simulink model "ES106A_StHlthSigStc"  (R2013b)
settings: Solver=FixedStepDiscrete  SolverMode=SingleTasking  StartTime=0.0  StopTime=1  FixedStep=0.002  RelTol=1e-3
values from neighbouring files (symbols this model uses):
  APPL10_CNT_U08 = DataDict.Constant    [ES106A_StHlthSigStc_DataDict.m]
  BITSPERBYTE_CNT_U08 = DataDict.Constant    [ES106A_StHlthSigStc_DataDict.m]
  ENOTOK_CNT_U08 = DataDict.Constant    [ES106A_StHlthSigStc_DataDict.m]
  EOK_CNT_U08 = DataDict.Constant    [ES106A_StHlthSigStc_DataDict.m]
  LOWRMASKVAL_CNT_U32 = DataDict.Constant    [ES106A_StHlthSigStc_DataDict.m]
  NROFCRCAREA_CNT_U08 = DataDict.ConfigParam    [ES106A_StHlthSigStc_DataDict.m]
  NVMAVRGPOSN_CNT_U08 = DataDict.Constant    [ES106A_StHlthSigStc_DataDict.m]
  NVMMAXPOSN_CNT_U08 = DataDict.Constant    [ES106A_StHlthSigStc_DataDict.m]
  NVMMINPOSN_CNT_U08 = DataDict.Constant    [ES106A_StHlthSigStc_DataDict.m]
  NVMSAMPLECNTRPOSN_CNT_U08 = DataDict.Constant    [ES106A_StHlthSigStc_DataDict.m]
  RAMAVRGPOSN_CNT_U08 = DataDict.Constant    [ES106A_StHlthSigStc_DataDict.m]
  RAMMAXPOSN_CNT_U08 = DataDict.Constant    [ES106A_StHlthSigStc_DataDict.m]
  RAMMINPOSN_CNT_U08 = DataDict.Constant    [ES106A_StHlthSigStc_DataDict.m]
  RAMRAWPOSN_CNT_U08 = DataDict.Constant    [ES106A_StHlthSigStc_DataDict.m]
  SIGCNT_ULS_U08 = DataDict.ConfigParam    [ES106A_StHlthSigStc_DataDict.m]
  SigStcPrmInst = DataDict.PIM    [ES106A_StHlthSigStc_DataDict.m]
  STHLTHMAXVAL_CNT_U08 = DataDict.Constant    [ES106A_StHlthSigStc_DataDict.m]
  WORDSIZE_CNT_U08 = DataDict.Constant    [ES106A_StHlthSigStc_DataDict.m]
undefined symbols (not defined in the file or in its folder): NvmGetErrSts1, StHlthTaskRef1
libraries: simulink x37, NxtrNvM x4, NxtrMax x4, NxtrMin x4
(part 5 of 5)

== system ES106A_StHlthSigStc/StHlthSigStc/StHlthStcPwrDwn/For Iterator Subsystem/If Action Subsystem/Statistical data computation for Controller Life Cycle/While Iterator Subsystem/Switch Case Action Subsystem ==
  In1 : Inport
  Action Port : ActionPort  ActionType=case
  CopyRight2 : Subsystem  Description=|  mask(Copyright Information){none=on}
      | Copyright info block.                                               
      |                                                                     
      | Place copyright information at the top of every subsystem in design.
      mask prompts: none "No parameters"
      mask help: Place copyright information at the top of every subsystem in design.
      mask Display:
      | NxtrConf = 'Nexteer Confidential';
      | 
      | sys = bdroot; %handle for the current model ("system")
      | first = get_param(sys,'Created');
      | if(isempty(first))
      |     first = datestr(now,'yyyy');
      | else
      |     first = first(end-3:end);  %year is last four digits
      | end
      | 
      | last = get_param(sys,'LastModifiedDate');
      | if isempty(last)
      |     last = datestr(now,'yyyy');
      | else
      |     last = last(end-3:end);
      | end
      | 
      | if strcmp(first,last)
      |     fprintf('%s -- Copyright %s Nexteer',NxtrConf,first)
      | else
      |     fprintf('%s -- %s%s- %s Nexteer',NxtrConf,char(169),first,last)
      | end
  Data Type Conversion : DataTypeConversion  OutDataTypeStr=uint32
  Shift Arithmetic3 : ArithShift  BitShiftNumber=SHIFTFAC24_ULS_U08  BitShiftDirection=Left
  Out1 : Outport
  wires:
  In1/1 -> Data Type Conversion/1
  Data Type Conversion/1 -> Shift Arithmetic3/1
  Shift Arithmetic3/1 -> Out1/1

== system ES106A_StHlthSigStc/StHlthSigStc/StHlthStcPwrDwn/For Iterator Subsystem/If Action Subsystem/Statistical data computation for Controller Life Cycle/While Iterator Subsystem/Switch Case Action Subsystem1 ==
  In1 : Inport
  Action Port : ActionPort  ActionType=case
  CopyRight2 : Subsystem  Description=|  mask(Copyright Information){none=on}
      | Copyright info block.                                               
      |                                                                     
      | Place copyright information at the top of every subsystem in design.
      mask prompts: none "No parameters"
      mask help: Place copyright information at the top of every subsystem in design.
      mask Display:
      | NxtrConf = 'Nexteer Confidential';
      | 
      | sys = bdroot; %handle for the current model ("system")
      | first = get_param(sys,'Created');
      | if(isempty(first))
      |     first = datestr(now,'yyyy');
      | else
      |     first = first(end-3:end);  %year is last four digits
      | end
      | 
      | last = get_param(sys,'LastModifiedDate');
      | if isempty(last)
      |     last = datestr(now,'yyyy');
      | else
      |     last = last(end-3:end);
      | end
      | 
      | if strcmp(first,last)
      |     fprintf('%s -- Copyright %s Nexteer',NxtrConf,first)
      | else
      |     fprintf('%s -- %s%s- %s Nexteer',NxtrConf,char(169),first,last)
      | end
  Data Type Conversion1 : DataTypeConversion  OutDataTypeStr=uint32
  Shift Arithmetic1 : ArithShift  BitShiftNumber=SHIFTFAC16_ULS_U08  BitShiftDirection=Left
  Out1 : Outport
  wires:
  In1/1 -> Data Type Conversion1/1
  Shift Arithmetic1/1 -> Out1/1
  Data Type Conversion1/1 -> Shift Arithmetic1/1

== system ES106A_StHlthSigStc/StHlthSigStc/StHlthStcPwrDwn/For Iterator Subsystem/If Action Subsystem/Statistical data computation for Controller Life Cycle/While Iterator Subsystem/Switch Case Action Subsystem2 ==
  In1 : Inport
  Action Port : ActionPort  ActionType=case
  CopyRight2 : Subsystem  Description=|  mask(Copyright Information){none=on}
      | Copyright info block.                                               
      |                                                                     
      | Place copyright information at the top of every subsystem in design.
      mask prompts: none "No parameters"
      mask help: Place copyright information at the top of every subsystem in design.
      mask Display:
      | NxtrConf = 'Nexteer Confidential';
      | 
      | sys = bdroot; %handle for the current model ("system")
      | first = get_param(sys,'Created');
      | if(isempty(first))
      |     first = datestr(now,'yyyy');
      | else
      |     first = first(end-3:end);  %year is last four digits
      | end
      | 
      | last = get_param(sys,'LastModifiedDate');
      | if isempty(last)
      |     last = datestr(now,'yyyy');
      | else
      |     last = last(end-3:end);
      | end
      | 
      | if strcmp(first,last)
      |     fprintf('%s -- Copyright %s Nexteer',NxtrConf,first)
      | else
      |     fprintf('%s -- %s%s- %s Nexteer',NxtrConf,char(169),first,last)
      | end
  Data Type Conversion1 : DataTypeConversion  OutDataTypeStr=uint32
  Shift Arithmetic2 : ArithShift  BitShiftNumber=SHIFTFAC8_ULS_U08  BitShiftDirection=Left
  Out1 : Outport
  wires:
  In1/1 -> Data Type Conversion1/1
  Data Type Conversion1/1 -> Shift Arithmetic2/1
  Shift Arithmetic2/1 -> Out1/1

== system ES106A_StHlthSigStc/StHlthSigStc/StHlthStcPwrDwn/For Iterator Subsystem/If Action Subsystem/Statistical data computation for Controller Life Cycle/While Iterator Subsystem/Switch Case Action Subsystem3 ==
  In1 : Inport
  Action Port : ActionPort  ActionType=case
  CopyRight2 : Subsystem  Description=|  mask(Copyright Information){none=on}
      | Copyright info block.                                               
      |                                                                     
      | Place copyright information at the top of every subsystem in design.
      mask prompts: none "No parameters"
      mask help: Place copyright information at the top of every subsystem in design.
      mask Display:
      | NxtrConf = 'Nexteer Confidential';
      | 
      | sys = bdroot; %handle for the current model ("system")
      | first = get_param(sys,'Created');
      | if(isempty(first))
      |     first = datestr(now,'yyyy');
      | else
      |     first = first(end-3:end);  %year is last four digits
      | end
      | 
      | last = get_param(sys,'LastModifiedDate');
      | if isempty(last)
      |     last = datestr(now,'yyyy');
      | else
      |     last = last(end-3:end);
      | end
      | 
      | if strcmp(first,last)
      |     fprintf('%s -- Copyright %s Nexteer',NxtrConf,first)
      | else
      |     fprintf('%s -- %s%s- %s Nexteer',NxtrConf,char(169),first,last)
      | end
  Data Type Conversion1 : DataTypeConversion  OutDataTypeStr=uint32
  Out1 : Outport
  wires:
  In1/1 -> Data Type Conversion1/1
  Data Type Conversion1/1 -> Out1/1

== system ES106A_StHlthSigStc/StHlthSigStc/StHlthStcPwrDwn/For Iterator Subsystem/If Action Subsystem/Update Nvm/Subsystem/CopyRight2 ==

== system ES106A_StHlthSigStc/StHlthSigStc/UpdStHlthStcData/Call Non Trusted Function /For Iterator Subsystem/Subsystem2/If Action Subsystem/CopyRight2 ==

== system ES106A_StHlthSigStc/StHlthSigStc/UpdStHlthStcData/Call Non Trusted Function /For Iterator Subsystem/Subsystem2/UpdateRamBuf/CopyRight2 ==

== system ES106A_StHlthSigStc/StHlthSigStc/UpdStHlthStcData/UpdDataSample/For Iterator Subsystem/Subsystem2/If Action Subsystem/CopyRight2 ==

== system ES106A_StHlthSigStc/StHlthSigStc/UpdStHlthStcData/UpdDataSample/For Iterator Subsystem/Subsystem2/UpdateRamBuf/CopyRight2 ==

== system ES106A_StHlthSigStc/StHlthSigStc/GetSigStcHlthData/If Action Subsystem1/GetSigStcHlthData/If Action Subsystem/While Iterator Subsystem/Switch Case Action Subsystem/CopyRight2 ==

== system ES106A_StHlthSigStc/StHlthSigStc/GetSigStcHlthData/If Action Subsystem1/GetSigStcHlthData/If Action Subsystem/While Iterator Subsystem/Switch Case Action Subsystem1/CopyRight2 ==

== system ES106A_StHlthSigStc/StHlthSigStc/GetSigStcHlthData/If Action Subsystem1/GetSigStcHlthData/If Action Subsystem/While Iterator Subsystem/Switch Case Action Subsystem2/CopyRight2 ==

== system ES106A_StHlthSigStc/StHlthSigStc/GetSigStcHlthData/If Action Subsystem1/GetSigStcHlthData/If Action Subsystem/While Iterator Subsystem/Switch Case Action Subsystem3/CopyRight2 ==

== system ES106A_StHlthSigStc/StHlthSigStc/StHlthStcPwrDwn/For Iterator Subsystem/If Action Subsystem/Statistical data computation for Controller Life Cycle/While Iterator Subsystem/Switch Case Action Subsystem/CopyRight2 ==

== system ES106A_StHlthSigStc/StHlthSigStc/StHlthStcPwrDwn/For Iterator Subsystem/If Action Subsystem/Statistical data computation for Controller Life Cycle/While Iterator Subsystem/Switch Case Action Subsystem1/CopyRight2 ==

== system ES106A_StHlthSigStc/StHlthSigStc/StHlthStcPwrDwn/For Iterator Subsystem/If Action Subsystem/Statistical data computation for Controller Life Cycle/While Iterator Subsystem/Switch Case Action Subsystem2/CopyRight2 ==

== system ES106A_StHlthSigStc/StHlthSigStc/StHlthStcPwrDwn/For Iterator Subsystem/If Action Subsystem/Statistical data computation for Controller Life Cycle/While Iterator Subsystem/Switch Case Action Subsystem3/CopyRight2 ==
